simulink model "HPF_model"  (R2020a)
settings: Solver=VariableStepAuto  StartTime=0.0  StopTime=0.1  RelTol=1e-3
values from neighbouring files (symbols this model uses):
  f = 100    [startup.m]
settings Model: Creator=Viraj  LastModifiedBy=Viraj

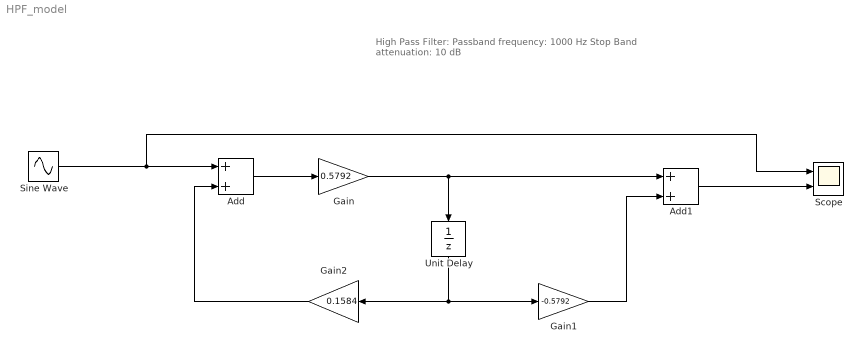
== system HPF_model ==
  note: High Pass Filter:
      | Passband frequency: 1000 Hz
      | Stop Band attenuation: 10 dB
  Add : Sum
  Add1 : Sum
  Gain : Gain  Gain=0.5792
  Gain1 : Gain  Gain=-0.5792
  Gain2 : Gain  Gain=0.1584
  Scope : Scope  NumInputPorts=2
  Sine Wave : Sin  Frequency=f*2*pi  SampleTime=1/(5000)
  Unit Delay : UnitDelay  SampleTime=-1  HasFrameUpgradeWarning=on
  wires:
  Add/1 -> Gain/1
  Gain/1 -> Unit Delay/1, Add1/1
  Unit Delay/1 -> Gain1/1, Gain2/1
  Gain1/1 -> Add1/2
  Gain2/1 -> Add/2
  Add1/1 -> Scope/2
  Sine Wave/1 -> Scope/1, Add/1
